simulink model "WindTurbine"  (Simulink 10.3)
settings: Solver=ode3  StartTime=0.0  StopTime=40  FixedStep=0.001  RelTol=1e-3
undefined symbols (not defined in the file): F, find_system, Fnom, gcbh, H, Llr, Lls, p, Pnom, Rr, Rs, sps_rtmsupport, Vnom, Wind_On
libraries: spsGroundLib x2, spsThreePhaseSeriesRLCLoadLib x2, spsThreePhaseVIMeasurementLib x2, spsThreePhaseBreakerLib x2, spsSeriesRLCBranchLib x1, spsPowerPhasorLib x1, simulink x1, spsThreePhaseProgrammableVoltageSourceLib x1, spsThreePhaseTransformerTwoWindingsLib x1, spsAsynchronousMachinepuUnitsLib x1, spsBistableLib x1, spsPower3phPhasorLib x1
settings Model: Creator=Redwan  LastModifiedBy=HP  MultithreadedSim=on
settings DataIOCC: SaveFormat=Dataset  SignalLoggingSaveFormat=Dataset
settings OptimizationCC: ExpressionDepthLimit=128  LifeSpan=auto
settings DebuggingCC: UnderspecifiedInitializationDetection=Simplified  MergeDetectMultiDrivingBlocksExec=error  FcnCallInpInsideContextMsg=error  StateNameClashWarn=none  SFUnexpectedBacktrackingDiag=error  SFNoUnconditionalDefaultTransitionDiag=error  SFExecutionAtInitializationDiag=warning
settings HardwareCC: ProdBitPerPointer=64  ProdBitPerSizeT=64  ProdBitPerPtrDiffT=64  ProdLargestAtomicFloat=Float  ProdIntDivRoundTo=Zero  ProdEndianess=LittleEndian  ProdWordSize=64  ProdHWDeviceType=Intel->x86-64 (Windows64)
settings ModelReferenceCC: PropagateSignalLabelsOutOfModel=on
settings CodeAppCC: StateflowObjectComments=off
settings GRTTargetCC: TargetLangStandard=C99 (ISO)  CombineOutputUpdateFcns=on  GRTInterface=off
settings ConfigComp: CovMetricSettings=dwe  CovSaveCumulativeToWorkspaceVar=off  CovSaveSingleToWorkspaceVar=off  CovExternalEMLEnable=on

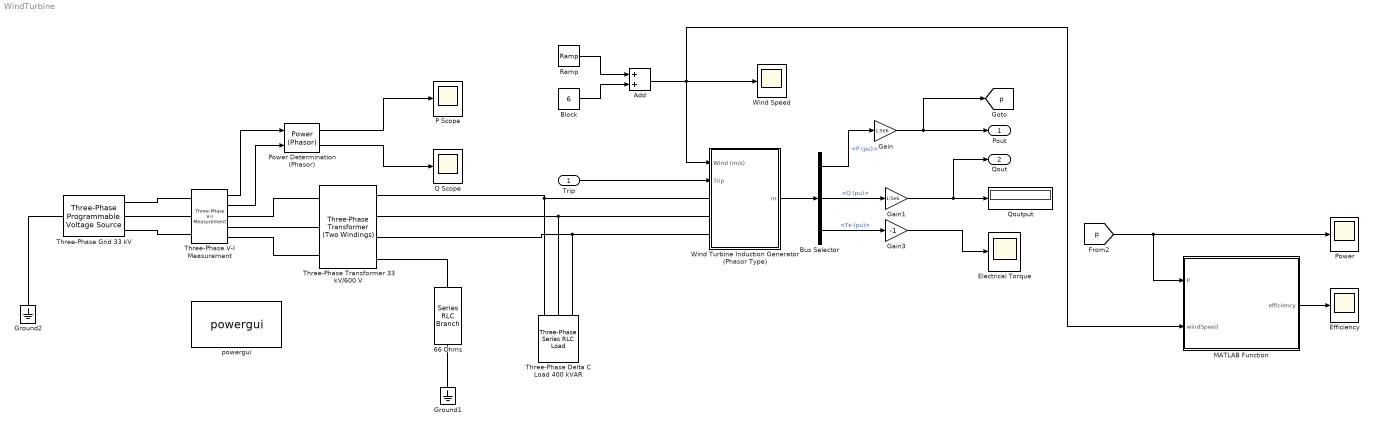
== system WindTurbine ==
  Trip : Inport
  "66 Ohms " : spsSeriesRLCBranchLib/Series RLC Branch  LConnTagsString=__new0  RConnTagsString=__new0  BranchType=R  Resistance=20  Inductance=1e-3  SetiL0=off  InitialCurrent=0  Capacitance=1e-6  Setx0=off  InitialVoltage=0  Measurements=None
  Add : Sum
  Block : Constant  Value=6
  Bus Selector : BusSelector  OutputSignals=P (pu),Q (pu),Te (pu)
  Efficiency : Scope
  Electrical Torque : Scope
  Gain : Gain  Gain=1.5e6
  Gain1 : Gain  Gain=1.5e6
  Gain3 : Gain  Gain=-1
  Ground1 : spsGroundLib/Ground  LConnTagsString=a
  Ground2 : spsGroundLib/Ground  LConnTagsString=a
  MATLAB Function : MATLAB Function  TreatAsAtomicUnit=on
  P Scope : Scope
  Power : Scope
  Power Determination (Phasor) : spsPowerPhasorLib/Power (Phasor)
      settings: SourceProductBaseCode=PS
  Q Scope : Scope
  "Qoutput " : Display
  Ramp : simulink/Sources/Ramp  slope=1  start=0  InitialOutput=0
  Three-Phase Delta C Load 400 kVAR : spsThreePhaseSeriesRLCLoadLib/Three-Phase Series RLC Load  LConnTagsString=A|B|C  Configuration=Delta  NominalVoltage=600  Vabc=[1e3 1e3 1e3]  Vabcp=[1e3 1e3 1e3]  NominalFrequency=50  UnbalancedPower=off  ActivePower=0  InductivePower=0  CapacitivePower=400e3  Pabc=[10e3 9e3 11e3]  QLabc=[100 90 110]  QCabc=[100 90 110]  Pabcp=[10e3 9e3 11e3]  QLabcp=[100 90 110]  QCabcp=[100 90 110]  Measurements=None  LoadType=constant Z
  Three-Phase Grid 33 kV : spsThreePhaseProgrammableVoltageSourceLib/Three-Phase Programmable Voltage Source  PositiveSequence="[33e3  0 50]"  VariationEntity=None  VariationType=Table of time-amplitude pairs  VariationTypeAlt=Step  VariationStep=0.5  VariationRate=10  VariationMagnitude=0.3  VariationFrequency=2  VariationTiming=[1 2]  VariationPhaseA=off  Amplitudes=[1 0.8 1.2 1.0]  TimeValues=[0 0.1 0.15 0.2]  HarmonicGeneration=off  HarmonicA=[3 0.2 -25 0]  HarmonicB=[2 0.15 35 2]  Timing="[0.05  3]"  BusType=swing  Pref=0  Qref=0  Qmin=-inf  Qmax=inf
  Three-Phase Transformer 33 kV/600 V : spsThreePhaseTransformerTwoWindingsLib/Three-Phase Transformer (Two Windings)  Winding1Connection=Yg  Winding2Connection=Yn  CoreType=Three single-phase transformers  SetSaturation=off  Hysteresis=off  DataFile='hysteresis'  SetInitialFlux=off  Measurements=None  UNITS=pu  NominalPower=[4e6 , 50 ]  Winding1=[33e3 , 0.025/30 , 0.025 ]  Winding2=[ 600 , 0.025/30 , 0.025 ]  Rm=500  Lm=inf  L0=0.5  Saturation=[ 0,0 ; 0.0024,1.2 ; 1.0,1.52 ]  InitialFluxes=[ 0.8 , -0.8 , 0.7 ]  BreakLoop=off  DiscreteSolver=Trapezoidal iterative  DataType=off  TransfoNumber=1
  Three-Phase V-I Measurement : spsThreePhaseVIMeasurementLib/Three-Phase V-I Measurement  VoltageMeasurement=phase-to-phase  SetLabelV=off  LabelV=Vabc  Vpu=off  VpuLL=off  CurrentMeasurement=yes  SetLabelI=off  LabelI=Iabc  Ipu=off  Pbase=100e6  Vbase=500e3  OutputType=Complex  PhasorSimulation=on  PSBequivalent=0
  "Wind Speed " : Scope
  Wind Turbine Induction Generator (Phasor Type) : Subsystem  AncestorBlock=|  DialogController=POWERSYS.PowerSysDialog  LoadFcn=sps_rtmsupport('LoadFcn',gcbh); %find_system(gcs,'FollowLinks', 'on', 'LookUnderMasks', 'all');  StartFcn=sps_rtmsupport('StartFcn',gcbh);  StopFcn=sps_rtmsupport('StopFcn',gcbh);  mask(Wind Turbine Induction Generator (Phasor Type)){ExternalTm=off, nom=[1.5e6 , 600, 50], sta=[ 0.004843, 0.1248], rot=[ 0.004377, 0.1791], Lm=6.77, mec=[5.04, 0.01, 3], init=[ -0.01,0,   0,0,0,   0,0,0 ], pitch_angle=0, Pmec=1.5e6, wind_base=12, speed_nom=1, P_wind_base=1, K_pitch_gain=[5 25], pitch_max=45, pitch_rate=2}
      | spsWindTurbineInductionGeneratorPhasorTypeLib/Wind Turbine
      | Induction Generator
      | (Phasor Type)
      mask prompts: ExternalTm "External turbine (Tm mechanical torque input)"; nom "Nominal power, line-to-line voltage, frequency [Pn(VA), Vn(Vrms), fn(Hz)]:"; sta "Stator [Rs, Lls] (pu):"; rot "Rotor [Rr', Llr'] (pu):"; Lm "Magnetizing inductance Lm (pu):"; mec "Inertia constant, friction factor, and pairs of poles: [H(s), F(pu), p]"; init "Initial conditions [s, th(deg), ias, ibs, ics (pu), ph_as, ph_bs, ph_cs (pu)]:"; pitch_angle "Pitch angle beta used to display characteristics (beta >=0)  (deg):"; Pmec "Nominal wind turbine mechanical output power (W):"; wind_base "Base wind speed (m/s):"; speed_nom "Base rotational speed (pu of base generator speed):"; P_wind_base "Maximum power at base wind speed (pu of nominal mechanical power):"; K_pitch_gain "Pitch angle controller gain: [Kp Ki]"; pitch_max "Maximum pitch angle (deg):"; pitch_rate "Maximum rate of change of pitch angle (deg/s):"
      mask help: Implements a phasor model of a squirrel-cage induction generator driven by a wind turbine.
      mask init:
      | [Pnom,Vnom,Fnom,Rs,Lls,Rr,Llr,H,p,F,Wind_On,FACTSroot] = WindTurbineIndGenInit (nom,sta,rot,mec,ExternalTm,wind_base,gcbh);
      settings: CopyFcn=sps_rtmsupport('CopyFcn',gcbh);  DeleteFcn=sps_rtmsupport('DeleteFcn',gcbh);  UndoDeleteFcn=sps_rtmsupport('UndoDeleteFcn',gcbh);  ModelCloseFcn=sps_rtmsupport('ModelCloseFcn',gcbh);  PreSaveFcn=sps_rtmsupport('PreSaveFcn',gcbh);  PostSaveFcn=sps_rtmsupport('PostSaveFcn',gcbh);  NameChangeFcn=sps_rtmsupport('NameChangeFcn',gcbh);  PreCopyFcn=sps_rtmsupport('PreCopyFcn',gcbh);  OpenFcn=sps_rtmsupport('OpenFcn',gcbh, [1]);  CloseFcn=sps_rtmsupport('CloseFcn',gcbh);  PreDeleteFcn=sps_rtmsupport('PreDeleteFcn',gcbh);
      mask Help: helpview(psbhelp);
      mask Callback ExternalTm: WindTurbineIndGenCback(gcbh);
      mask DialogControl display Prompt: Display wind turbine power characteristics
      mask DialogControl display Callback: WindTurbineIndGenDisplay(gcbh);
      mask Display:
      | port_label('LConn',1,'A')
      | port_label('LConn',2,'B')
      | port_label('LConn',3,'C')
      | port_label('output',1,'m')
      | switch get_param(gcbh,'ExternalTm')
      |     case 'on'
      |         port_label('input',1,'Tm')
      |     case 'off'
      |         port_label('input',1,'wind')
      | end
      | port_label('input',2,'trip')
  powergui : spspowerguiLib/powergui  Priority=1  SimulationMode=Phasor  SampleTime=50e-6  frequency=50  Iterations=50  frequencyindice=50  Pbase=100e6  ErrMax=1e-4  UnitsV=V  UnitsW=W  buscounter=0  FunctionMessages=off  echomessages=off  EnableUseOfTLC=off  CurrentSourceSwitches=off  DisableSnubberDevices=off  DisableRonSwitches=off  DisableVfSwitches=off  DisplayEquations=off  AutomaticDiscreteSolvers=off  SolverType=Tustin/Backward Euler (TBE)  Interpol=off  ExternalGateDelay=off  methode=off  Ts=100  x0status=blocks  SPID=on  SwTol=0  HookPort=off  NonlinearTolerance=1e-4  nMaxIteration=100  ContinueOnMaxIteration=off  RestoreLinks=warning  ResistiveCurrentMeasurement=off  Frange=[0:2:500]  Ylog=off  Xlog=on  ShowGrid=off  save=off  variable=ZData  structure=0  ZoomFFT=off  StartTime=0.0  cycles=1  DisplayStyle=1  fundamental=60  FreqAxis=off  MaxFrequency=1000  frequencyindicesteady=1  RmsSteady=1  display=off
  Pout : Outport  VectorParamsAs1DForOutWhenUnconnected=off
  Qout : Outport  Port=2  VectorParamsAs1DForOutWhenUnconnected=off
  tag scope: p=global
  wires:
  Trip/1 -> Wind Turbine Induction Generator (Phasor Type)/2(Trip)
  Gain/1 -> [p], Pout/1
  Gain1/1 -> Qout/1, "Qoutput "/1
  Bus Selector/2 -> Gain1/1  "<Q (pu)>"
  Wind Turbine Induction Generator (Phasor Type)/1(m) -> Bus Selector/1
  Ramp/1 -> Add/1
  Block/1 -> Add/2
  Add/1 -> Wind Turbine Induction Generator (Phasor Type)/1("Wind (m/s) "), MATLAB Function/2(windSpeed), "Wind Speed "/1
  Power Determination (Phasor)/2 -> Q Scope/1
  Power Determination (Phasor)/1 -> P Scope/1
  Three-Phase V-I Measurement/1 -> Power Determination (Phasor)/1
  Three-Phase V-I Measurement/2 -> Power Determination (Phasor)/2
  [p] -> Power/1, MATLAB Function/1(P)
  MATLAB Function/1(efficiency) -> Efficiency/1
  Bus Selector/3 -> Gain3/1  "<Te (pu)>"
  Gain3/1 -> Electrical Torque/1
  Bus Selector/1 -> Gain/1  "<P (pu)>"
  connections:
  Ground1/LConn1 -- "66 Ohms "/RConn1
  Three-Phase Transformer 33 kV/600 V/RConn4 -- "66 Ohms "/LConn1
  Three-Phase Grid 33 kV/LConn1 -- Ground2/LConn1
  Three-Phase Transformer 33 kV/600 V/RConn1 -- Three-Phase Delta C Load 400 kVAR/LConn1 -- Wind Turbine Induction Generator (Phasor Type)/LConn1
  Three-Phase Transformer 33 kV/600 V/RConn2 -- Three-Phase Delta C Load 400 kVAR/LConn2 -- Wind Turbine Induction Generator (Phasor Type)/LConn2
  Three-Phase Transformer 33 kV/600 V/RConn3 -- Wind Turbine Induction Generator (Phasor Type)/LConn3 -- Three-Phase Delta C Load 400 kVAR/LConn3
  Three-Phase Grid 33 kV/RConn1 -- Three-Phase V-I Measurement/LConn1
  Three-Phase Grid 33 kV/RConn2 -- Three-Phase V-I Measurement/LConn2
  Three-Phase Grid 33 kV/RConn3 -- Three-Phase V-I Measurement/LConn3
  Three-Phase V-I Measurement/RConn1 -- Three-Phase Transformer 33 kV/600 V/LConn1
  Three-Phase V-I Measurement/RConn2 -- Three-Phase Transformer 33 kV/600 V/LConn2
  Three-Phase V-I Measurement/RConn3 -- Three-Phase Transformer 33 kV/600 V/LConn3

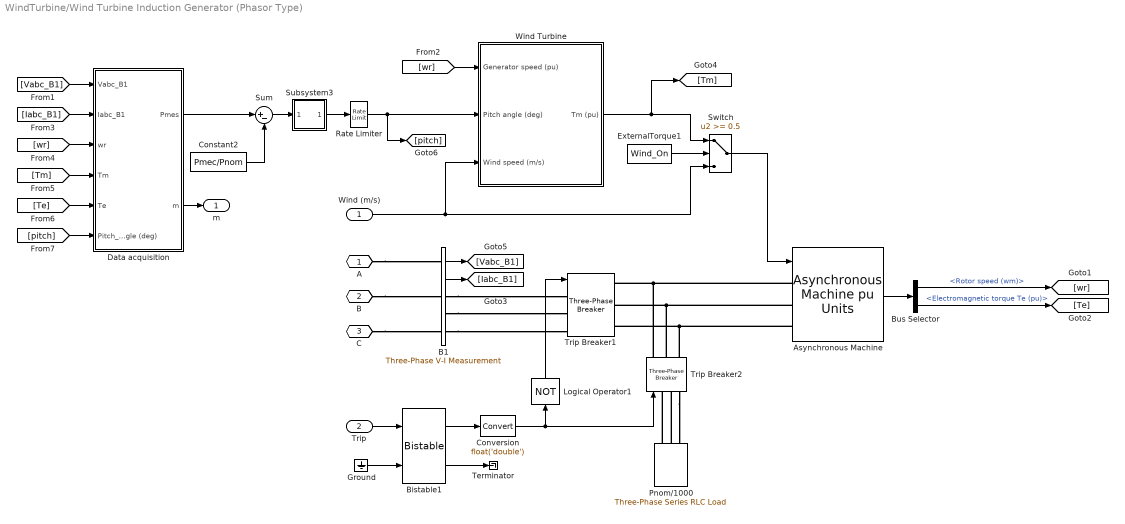
== system WindTurbine/Wind Turbine Induction Generator (Phasor Type) ==
  "Wind (m/s) " : Inport
  Trip : Inport  Port=2
  Asynchronous Machine : spsAsynchronousMachinepuUnitsLib/Asynchronous Machine pu Units  RotorType=Squirrel-cage  PresetModel=No  MechanicalLoad=Torque Tm  ShowDetailedParameters=on  ReferenceFrame=Rotor  Units=pu  MeasurementBus=off  NominalParameters=[ Pnom Vnom Fnom ]  VoltageRatio=1  Stator=[ Rs Lls]  Rotor=[ Rr Llr]  Cage1=[0.01909 0.0397]  Cage2=[0.01909 0.0397]  Lm=Lm  Mechanical=[H F p]  PolePairs=3  InitialConditions=init  SimulateSaturation=off  Saturation=[ 0 0 ; 0 0 ]  LoadFlowParameters=0  TsPowergui=0  TsBlock=-1  IterativeModel=Forward Euler  IterativeDiscreteModel=Trapezoidal non iterative  Pmec=0
      settings: SourceProductBaseCode=PS
  B1 : spsThreePhaseVIMeasurementLib/Three-Phase V-I Measurement  VoltageMeasurement=phase-to-ground  SetLabelV=off  LabelV=Vabc_B1  Vpu=on  VpuLL=off  CurrentMeasurement=yes  SetLabelI=off  LabelI=Iabc_Beol  Ipu=on  Pbase=Pnom  Vbase=Vnom  OutputType=Complex  PhasorSimulation=on  PSBequivalent=0
  Bistable1 : spsBistableLib/Bistable  Qpriority=Set  ic=0  Ts=0
      settings: SourceProductBaseCode=PS
  Bus Selector : BusSelector  OutputSignals=Mechanical.Rotor speed (wm),Mechanical.Electromagnetic torque Te (pu)
  Constant2 : Constant  Value=Pmec/Pnom
  Conversion : DataTypeConversion  OutDataTypeStr=float('double')
  Data acquisition : Subsystem
  ExternalTorque1 : Constant  Value=Wind_On
  Ground : Ground
  Logical Operator1 : Logic  Operator=NOT  AllPortsSameDT=off  OutDataTypeStr=float('double')  SampleTime=0
  Pnom/1000 : spsThreePhaseSeriesRLCLoadLib/Three-Phase Series RLC Load  LConnTagsString=A|B|C  Configuration=Y (grounded)  NominalVoltage=Vnom  Vabc=[1e3 1e3 1e3]  Vabcp=[1e3 1e3 1e3]  NominalFrequency=Fnom  UnbalancedPower=off  ActivePower=Pnom/1000  InductivePower=0  CapacitivePower=0  Pabc=[10e3 9e3 11e3]  QLabc=[100 90 110]  QCabc=[100 90 110]  Pabcp=[10e3 9e3 11e3]  QLabcp=[100 90 110]  QCabcp=[100 90 110]  Measurements=None  LoadType=constant Z
  "Rate Limiter   " : RateLimiter  RisingSlewLimit=pitch_rate  FallingSlewLimit=-pitch_rate
  Subsystem3 : Subsystem  mask{Kp=K_pitch_gain(1), Ki=K_pitch_gain(2), Limits=[pitch_max 0], Init=0}
      mask prompts: Kp "Proportional gain (Kp):"; Ki "Integral gain (Ki):"; Limits "Output limits [Upper Lower]:"; Init "Output initial value:"
      mask init:
      | Upper_Limit=Limits(1);
      | Lower_Limit=Limits(2);
      mask Display: disp('PI')
  Sum : Sum  Inputs=|+-  SaturateOnIntegerOverflow=on
  Switch : Switch  Threshold=0.5  SaturateOnIntegerOverflow=on
  Terminator : Terminator
  Trip Breaker1 : spsThreePhaseBreakerLib/Three-Phase Breaker  InitialState=closed  SwitchA=on  SwitchB=on  SwitchC=on  SwitchTimes="[4/60  10/60]"  External=on  BreakerResistance=0.001  SnubberResistance=1e6  SnubberCapacitance=inf  Measurements=None
  Trip Breaker2 : spsThreePhaseBreakerLib/Three-Phase Breaker  InitialState=open  SwitchA=on  SwitchB=on  SwitchC=on  SwitchTimes="[4/60  10/60]"  External=on  BreakerResistance=0.001  SnubberResistance=1e6  SnubberCapacitance=inf  Measurements=None
  Wind Turbine : Subsystem  AncestorBlock=spsWindTurbineLib/Wind Turbine  DialogController=POWERSYS.PowerSysDialog  mask(Wind Turbine){Pnom=Pmec, Pelec_base=Pnom, wind_base=wind_base, P_wind_base=P_wind_base, speed_nom=speed_nom, pitch_angle=0, c1_c6=[0.51763          116          0.4            5           21     0.006795], cp_nom=0.48, lambda_nom=8.1}
      mask prompts: Pnom "Nominal mechanical output power (W):"; Pelec_base "Base power of the electrical generator (VA):"; wind_base "Base wind speed (m/s):"; P_wind_base "Maximum power at base wind speed (pu of nominal mechanical power):"; speed_nom "Base rotational speed (p.u. of base generator speed):"; pitch_angle "Pitch angle beta to display wind-turbine power characteristics (beta >=0)  (deg):"
      mask help:
      | This block implements a variable pitch wind turbine model. The performance coefficient Cp of the turbine is the mechanical output power of the turbine divided by wind power and a function of wind speed, rotational speed, and pitch angle (beta). Cp reaches its maximum value at zero beta. Select the wind-turbine power characteristics display to plot the turbine characteristics at the specified pitch angle.
      |
      | The first input is the generator speed in per unit of the generator base speed. For a synchronous or asynchronous generator, the base speed is the synchronous speed. For a permanent-magnet generator, the base speed is defined as the speed producing nominal voltage at  no load. The second input is the blade pitch angle (beta) in degrees. The third input is the wind speed in m/s.
      |
      | The output is the torque applied to the generator shaft in per unit of the generator ratings.
      |
      | The turbine inertia must be added to the generator inertia.
      mask init:
      | c1=c1_c6(1);c2=c1_c6(2);c3=c1_c6(3);c4=c1_c6(4);c5=c1_c6(5);c6=c1_c6(6);
      | 
      | if Pnom<=0
      |     error(message('physmod:powersys:common:GreaterThan',getfullname(gcbh),'Nominal mechanical output power',0));
      | end
      | if Pelec_base<=0
      |     error(message('physmod:powersys:common:GreaterThan',getfullname(gcbh),'Base power of the electrical generator',0));
      | end
      | if wind_base<=0
      |     error(message('physmod:powersys:common:GreaterThan',getfullname(gcbh),'Base wind speed (m/s)',0));
      | end
      | if P_wind_base<=0
      |     error(message('physmod:powersys:common:GreaterThan',getfullname(gcbh),'Maximum power at base wind speed',0));
      | end
      | power_initmask();
      settings: OpenFcn=sps_rtmsupport('OpenFcn',gcbh)
      mask Help: helpview(psbhelp);
      mask DialogControl DisplayTurbChar Prompt: Display wind turbine power characteristics
      mask DialogControl DisplayTurbChar Callback: WindTurbinePlot(gcb)
  A : PMIOPort  Side=Left
  B : PMIOPort  Port=2  Side=Left
  C : PMIOPort  Port=3  Side=Left
  m : Outport  VectorParamsAs1DForOutWhenUnconnected=off
  wires:
  [wr] -> Wind Turbine/1(Generator speed (pu))
  Data acquisition/1(Pmes) -> Sum/1
  Logical Operator1/1 -> Trip Breaker1/1
  Conversion/1 -> Trip Breaker2/1, Logical Operator1/1
  Constant2/1 -> Sum/2
  Subsystem3/1(Out1) -> "Rate Limiter   "/1
  Sum/1 -> Subsystem3/1(In1)
  Switch/1 -> Asynchronous Machine/1
  ExternalTorque1/1 -> Switch/2
  Bistable1/1 -> Conversion/1
  Ground/1 -> Bistable1/2
  Bistable1/2 -> Terminator/1
  Trip/1 -> Bistable1/1
  [pitch] -> Data acquisition/6(Pitch_angle (deg))
  [Te] -> Data acquisition/5(Te)
  [Tm] -> Data acquisition/4(Tm)
  [wr] -> Data acquisition/3(wr)
  [Vabc_B1] -> Data acquisition/1(Vabc_B1)
  [Iabc_B1] -> Data acquisition/2(Iabc_B1)
  Bus Selector/2 -> [Te]  "<Electromagnetic torque Te (pu)>"
  Bus Selector/1 -> [wr]  "<Rotor speed (wm)>"
  "Rate Limiter   "/1 -> [pitch], Wind Turbine/2(Pitch angle (deg))
  Data acquisition/2(m) -> m/1
  "Wind (m/s) "/1 -> Switch/3, Wind Turbine/3(Wind speed (m/s))
  B1/1 -> [Vabc_B1]
  B1/2 -> [Iabc_B1]
  Wind Turbine/1(Tm (pu)) -> [Tm], Switch/1
  Asynchronous Machine/1 -> Bus Selector/1
  connections:
  Pnom/1000/LConn2 -- Trip Breaker2/LConn2
  Pnom/1000/LConn1 -- Trip Breaker2/LConn1
  B1/RConn2 -- Trip Breaker1/LConn2
  B1/RConn1 -- Trip Breaker1/LConn1
  Asynchronous Machine/LConn3 -- Trip Breaker1/RConn3 -- Trip Breaker2/RConn3
  Asynchronous Machine/LConn2 -- Trip Breaker1/RConn2 -- Trip Breaker2/RConn2
  Asynchronous Machine/LConn1 -- Trip Breaker1/RConn1 -- Trip Breaker2/RConn1
  A/RConn1 -- B1/LConn1
  C/RConn1 -- B1/LConn3
  B/RConn1 -- B1/LConn2
  B1/RConn3 -- Trip Breaker1/LConn3
  Trip Breaker2/LConn3 -- Pnom/1000/LConn3

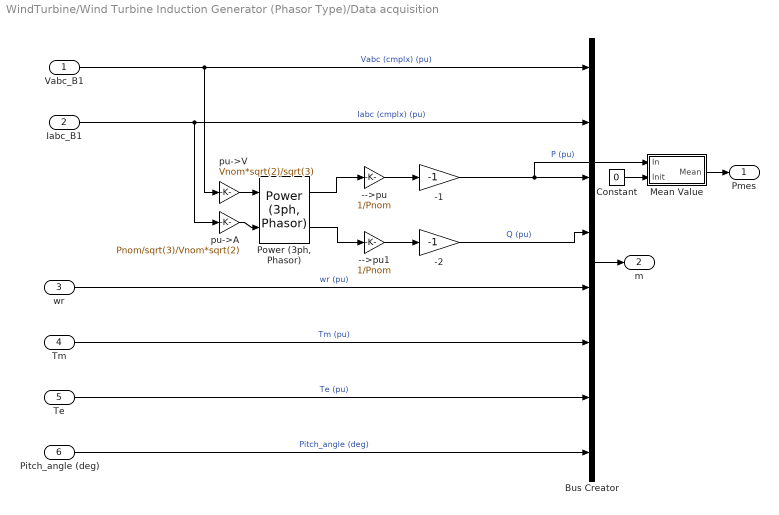
== system WindTurbine/Wind Turbine Induction Generator (Phasor Type)/Data acquisition ==
  Vabc_B1 : Inport
  Iabc_B1 : Inport  Port=2
  wr : Inport  Port=3
  Tm : Inport  Port=4
  Te : Inport  Port=5
  Pitch_angle (deg) : Inport  Port=6
  -->pu : Gain  Gain=1/Pnom  SaturateOnIntegerOverflow=on  OutDataTypeStr=Inherit: Same as input  ParamDataTypeStr=Inherit: Same as input
  -->pu1 : Gain  Gain=1/Pnom  SaturateOnIntegerOverflow=on  OutDataTypeStr=Inherit: Same as input  ParamDataTypeStr=Inherit: Same as input
  -1 : Gain  Gain=-1  SaturateOnIntegerOverflow=on  OutDataTypeStr=Inherit: Same as input  ParamDataTypeStr=Inherit: Same as input
  -2 : Gain  Gain=-1  SaturateOnIntegerOverflow=on  OutDataTypeStr=Inherit: Same as input  ParamDataTypeStr=Inherit: Same as input
  Bus Creator : BusCreator  Inputs=8
  Constant : Constant  Value=0
  Mean Value : Subsystem  mask(Mean value){Period=1/Fnom}
      mask prompts: Period "Averaging period (s):"
      mask help: This block uses the running window averaging technique to compute the mean value of the input signal over the specified period.
  "Power (3ph, Phasor)" : spsPower3phPhasorLib/Power (3ph, Phasor)
      settings: SourceProductBaseCode=PS
  pu->A : Gain  Gain=Pnom/sqrt(3)/Vnom*sqrt(2)  SaturateOnIntegerOverflow=on  OutDataTypeStr=Inherit: Same as input  ParamDataTypeStr=Inherit: Same as input
  pu->V : Gain  Gain=Vnom*sqrt(2)/sqrt(3)  SaturateOnIntegerOverflow=on  OutDataTypeStr=Inherit: Same as input  ParamDataTypeStr=Inherit: Same as input
  Pmes : Outport  VectorParamsAs1DForOutWhenUnconnected=off
  m : Outport  Port=2  VectorParamsAs1DForOutWhenUnconnected=off
  wires:
  pu->A/1 -> "Power (3ph, Phasor)"/2
  -->pu/1 -> -1/1
  pu->V/1 -> "Power (3ph, Phasor)"/1
  -2/1 -> Bus Creator/4  "Q (pu)"
  -1/1 -> Mean Value/1(In), Bus Creator/3  "P (pu)"
  wr/1 -> Bus Creator/5  "wr (pu)"
  Tm/1 -> Bus Creator/6  "Tm (pu)"
  Te/1 -> Bus Creator/7  "Te (pu)"
  Pitch_angle (deg)/1 -> Bus Creator/8  "Pitch_angle (deg)"
  Vabc_B1/1 -> pu->V/1, Bus Creator/1  "Vabc (cmplx) (pu)"
  Iabc_B1/1 -> pu->A/1, Bus Creator/2  "Iabc (cmplx) (pu)"
  Constant/1 -> Mean Value/2(Init)
  Mean Value/1(Mean) -> Pmes/1
  Bus Creator/1 -> m/1
  -->pu1/1 -> -2/1
  "Power (3ph, Phasor)"/1 -> -->pu/1
  "Power (3ph, Phasor)"/2 -> -->pu1/1

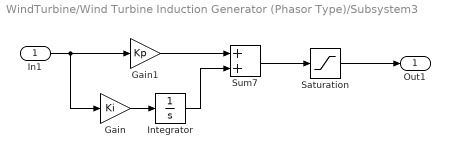
== system WindTurbine/Wind Turbine Induction Generator (Phasor Type)/Subsystem3 ==
  In1 : Inport
  Gain : Gain  Gain=Ki  SaturateOnIntegerOverflow=on  OutDataTypeStr=Inherit: Same as input  ParamDataTypeStr=Inherit: Same as input
  Gain1 : Gain  Gain=Kp  SaturateOnIntegerOverflow=on  OutDataTypeStr=Inherit: Same as input  ParamDataTypeStr=Inherit: Same as input
  Integrator : Integrator  InitialCondition=Init  LimitOutput=on  UpperSaturationLimit=Upper_Limit  LowerSaturationLimit=Lower_Limit
  Saturation : Saturate  UpperLimit=Upper_Limit  LowerLimit=Lower_Limit
  Sum7 : Sum  InputSameDT=on  SaturateOnIntegerOverflow=on  OutDataTypeStr=Inherit: Same as first input
  Out1 : Outport  VectorParamsAs1DForOutWhenUnconnected=off
  wires:
  Gain/1 -> Integrator/1
  Gain1/1 -> Sum7/1
  Integrator/1 -> Sum7/2
  In1/1 -> Gain1/1, Gain/1
  Sum7/1 -> Saturation/1
  Saturation/1 -> Out1/1

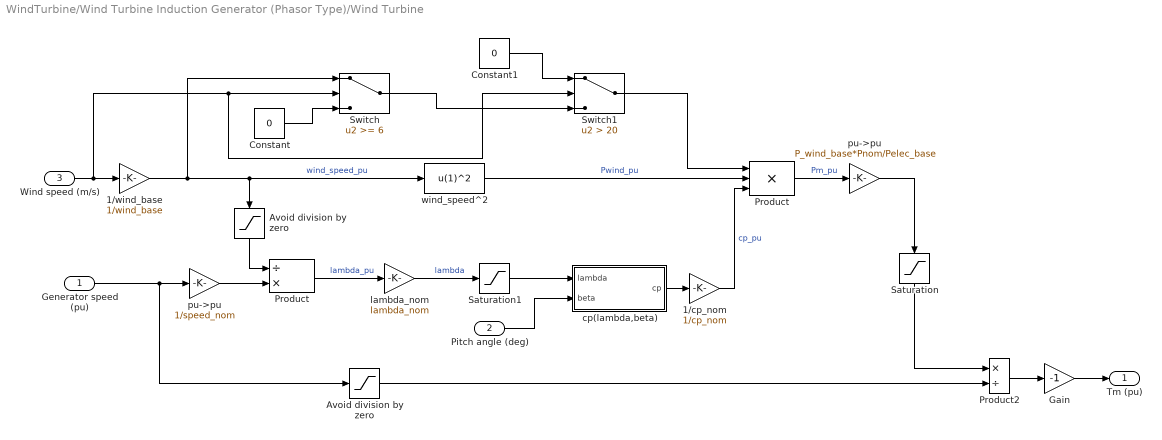
== system WindTurbine/Wind Turbine Induction Generator (Phasor Type)/Wind Turbine ==
  Generator speed (pu) : Inport
  Pitch angle (deg) : Inport  Port=2
  Wind speed (m/s) : Inport  Port=3
  1/cp_nom : Gain  Gain=1/cp_nom  SaturateOnIntegerOverflow=on  OutDataTypeStr=Inherit: Same as input  ParamDataTypeStr=Inherit: Same as input
  1/wind_base : Gain  Gain=1/wind_base  SaturateOnIntegerOverflow=on  OutDataTypeStr=Inherit: Same as input  ParamDataTypeStr=Inherit: Same as input
  Avoid division by zero : Saturate  UpperLimit=1e6  LowerLimit=1e-6
  "Avoid division by zero " : Saturate  UpperLimit=1e6  LowerLimit=1e-6
  Constant : Constant  Value=0
  Constant1 : Constant  Value=0
  Gain : Gain  Gain=-1  SaturateOnIntegerOverflow=on  OutDataTypeStr=Inherit: Same as input  ParamDataTypeStr=Inherit: Same as input
  Product : Product  Inputs=/*  SaturateOnIntegerOverflow=on  OutDataTypeStr=Inherit: Same as first input
  "Product " : Product  Inputs=3  SaturateOnIntegerOverflow=on  OutDataTypeStr=Inherit: Same as first input
  Product2 : Product  Inputs=*/  InputSameDT=on  SaturateOnIntegerOverflow=on  OutDataTypeStr=Inherit: Same as first input
  Saturation : Saturate  UpperLimit=1  LowerLimit=0  OutMin=[-0.5]  OutMax=[1]
  Saturation1 : Saturate  UpperLimit=inf  LowerLimit=1e-6
  Switch : Switch  Threshold=6
  Switch1 : Switch  Criteria=u2 > Threshold  Threshold=20
  cp(lambda,beta) : Subsystem
  lambda_nom : Gain  Gain=lambda_nom  SaturateOnIntegerOverflow=on  OutDataTypeStr=Inherit: Same as input  ParamDataTypeStr=Inherit: Same as input
  pu->pu : Gain  Gain=P_wind_base*Pnom/Pelec_base  SaturateOnIntegerOverflow=on  OutDataTypeStr=Inherit: Same as input  ParamDataTypeStr=Inherit: Same as input
  "pu->pu " : Gain  Gain=1/speed_nom  SaturateOnIntegerOverflow=on  OutDataTypeStr=Inherit: Same as input  ParamDataTypeStr=Inherit: Same as input
  wind_speed^2 : Fcn  Expr=u(1)^2
  Tm (pu) : Outport  VectorParamsAs1DForOutWhenUnconnected=off
  wires:
  "pu->pu "/1 -> Product/2
  "Avoid division by zero "/1 -> Product/1
  1/wind_base/1 -> Switch/1, "Avoid division by zero "/1, wind_speed^2/1  "wind_speed_pu"
  Product/1 -> lambda_nom/1  "lambda_pu"
  lambda_nom/1 -> Saturation1/1  "lambda"
  "Product "/1 -> pu->pu/1  "Pm_pu"
  Generator speed (pu)/1 -> "pu->pu "/1, Avoid division by zero/1
  Gain/1 -> Tm (pu)/1
  Wind speed (m/s)/1 -> Switch/2, Switch1/2, 1/wind_base/1
  Avoid division by zero/1 -> Product2/2
  Product2/1 -> Gain/1
  cp(lambda,beta)/1(cp) -> 1/cp_nom/1
  pu->pu/1 -> Saturation/1
  Pitch angle (deg)/1 -> cp(lambda,beta)/2(beta)
  Saturation1/1 -> cp(lambda,beta)/1(lambda)
  Constant/1 -> Switch/3
  Constant1/1 -> Switch1/1
  Switch/1 -> Switch1/3
  1/cp_nom/1 -> "Product "/3  "cp_pu"
  wind_speed^2/1 -> "Product "/2  "Pwind_pu"
  Switch1/1 -> "Product "/1
  Saturation/1 -> Product2/1

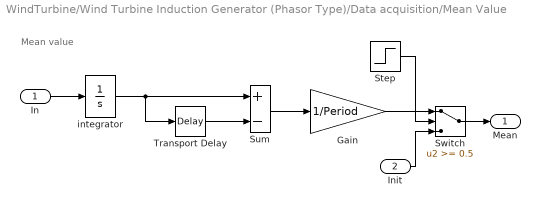
== system WindTurbine/Wind Turbine Induction Generator (Phasor Type)/Data acquisition/Mean Value ==
  note: Mean value
  In : Inport
  Init : Inport  Port=2
  Gain : Gain  Gain=1/Period  SaturateOnIntegerOverflow=on  OutDataTypeStr=Inherit: Same as input  ParamDataTypeStr=Inherit: Same as input
  Step : Step  Time=Period+eps  SampleTime=0
  Sum : Sum  Inputs=+-  InputSameDT=on  SaturateOnIntegerOverflow=on  OutDataTypeStr=Inherit: Same as first input
  Switch : Switch  Threshold=0.5  SaturateOnIntegerOverflow=on
  Transport Delay : TransportDelay  DelayTime=Period
  integrator : Integrator
  Mean : Outport  VectorParamsAs1DForOutWhenUnconnected=off
  wires:
  Init/1 -> Switch/3
  Step/1 -> Switch/2
  Switch/1 -> Mean/1
  Gain/1 -> Switch/1
  Sum/1 -> Gain/1
  In/1 -> integrator/1
  integrator/1 -> Sum/1, Transport Delay/1
  Transport Delay/1 -> Sum/2

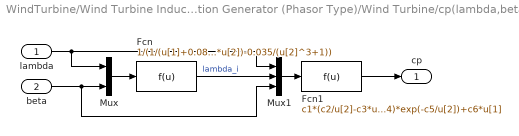
== system WindTurbine/Wind Turbine Induction Generator (Phasor Type)/Wind Turbine/cp(lambda,beta) ==
  lambda : Inport
  beta : Inport  Port=2
  Fcn : Fcn  Expr=1/(1/(u[1]+0.08*u[2])-0.035/(u[2]^3+1))
  Fcn1 : Fcn  Expr=c1*(c2/u[2]-c3*u[3]-c4)*exp(-c5/u[2])+c6*u[1]
  Mux : Mux  Inputs=2
  Mux1 : Mux  Inputs=3
  cp : Outport  VectorParamsAs1DForOutWhenUnconnected=off
  wires:
  Mux/1 -> Fcn/1
  beta/1 -> Mux/2, Mux1/3
  Mux1/1 -> Fcn1/1
  lambda/1 -> Mux/1, Mux1/1
  Fcn1/1 -> cp/1
  Fcn/1 -> Mux1/2  "lambda_i"

== matlab function MATLAB Function ==
  data: P input double; windSpeed input double; efficiency output double
function efficiency = Efficiency(P, windSpeed)
    rho = 1.29;
    Area = [2290.22 6647.61 13273.23];
    windPower = 0.5 * (windSpeed) ^ 3 * rho .* Area;
    efficiency = 100 * P ./ windPower;
end
